simulink model "DC_Mach1"  (Simulink 4.00)
settings: Solver=ode23tb  StartTime=0.0  StopTime=5  MaxStep=1e-3
InitFcn:
  | powericon('psbinitsys',bdroot);
libraries: powerlib2 x2
settings Model: LastModifiedBy=ieao  BlockReductionOpt=off

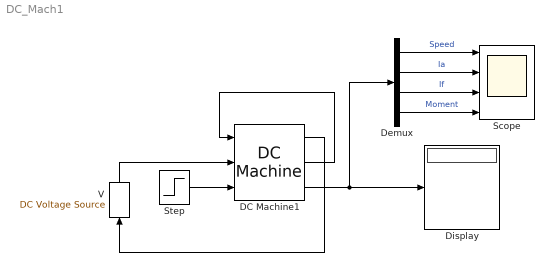
== system DC_Mach1 ==
  DC Machine1 : powerlib2/Machines/DC Machine  RLa="[ 2.52  0.048]"  RLf=[ 92 120]  Laf=0.207  J=0.01  Bm=0  Tf=0  w0=0  PSBOutputType=110
  Demux : Demux  Outputs=4  BusSelectionMode=off
  Display : Display
      settings: Format=short
  Scope : Scope  NumInputPorts=4
      settings: TimeRange=auto  YMin=0~3~3~0  YMax=900~8.5~8.5~15  SaveToWorkspace=off  SaveName=ScopeData  MaxDataPoints=5000
  Step : Step  Time=0.2  Before=0  After=2.378  SampleTime=0
  V : powerlib2/Electrical Sources/DC Voltage Source  Tag=PoWeRsYsTeMbLoCk  Description=source block  Orientation=up  V=800  mesure=None  PSBOutputType=1
  wires:
  V/1 -> DC Machine1/2
  DC Machine1/3 -> Display/1, Demux/1
  Step/1 -> DC Machine1/3
  DC Machine1/2 -> DC Machine1/1
  DC Machine1/1 -> V/1
  Demux/1 -> Scope/1  "Speed"
  Demux/2 -> Scope/2  "Ia"
  Demux/3 -> Scope/3  "If"
  Demux/4 -> Scope/4  "Moment"
